simulink model "Q5"  (R2017b)
settings: Solver=VariableStepAuto  StartTime=0.0  StopTime=50  RelTol=1e-3
libraries: simulink x2
settings Model: Creator=HeMaTshop  LastModifiedBy=HeMaTshop

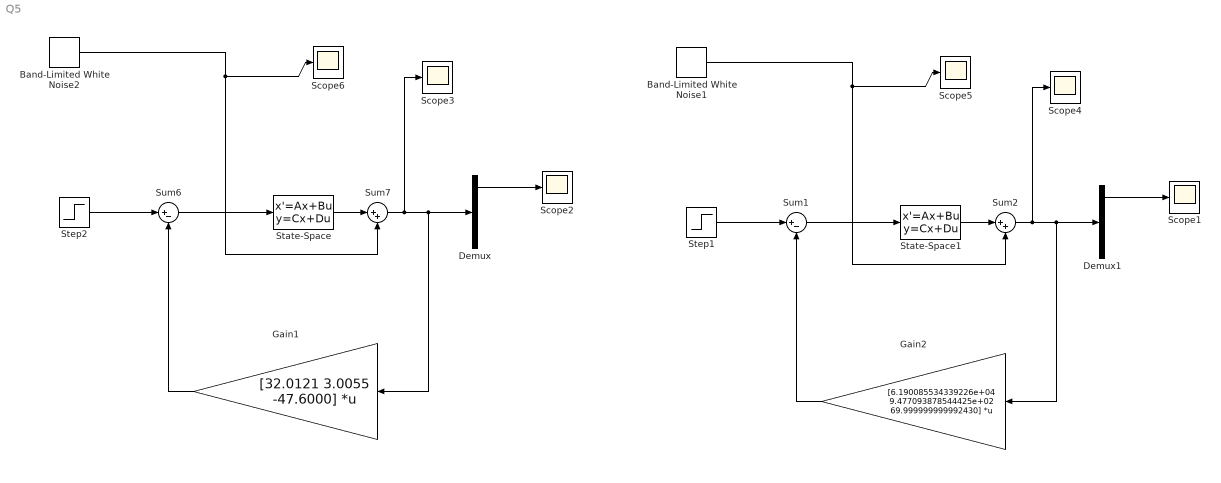
== system Q5 ==
  Band-Limited White Noise1 : simulink/Sources/Band-Limited White Noise  Cov=[0.001]  Ts=1  seed=[23341]
  Band-Limited White Noise2 : simulink/Sources/Band-Limited White Noise  Cov=[0.001]  Ts=1  seed=[23341]
  Demux : Demux  Outputs=3
  Demux1 : Demux  Outputs=3
  Gain1 : Gain  Gain="[32.0121    3.0055  -47.6000]"  Multiplication=Matrix(K*u)
  Gain2 : Gain  Gain="[6.190085534339226e+04    9.477093878544425e+02  69.999999999992430]"  Multiplication=Matrix(K*u)
  Scope{1..6} (6 alike) : Scope
  State-Space : StateSpace  A=[0 1 0;9.8/0.03 0 24.8656;0 0 -250]  B=[0;0;5]  C=eye(3)  D=[0;0;0]  InitialCondition=0
  State-Space1 : StateSpace  A=[0 1 0;9.8/0.03 0 24.8656;0 0 -250]  B=[0;0;5]  C=eye(3)  D=[0;0;0]  InitialCondition=0
  Step1 : Step  Time=0  SampleTime=0
  Step2 : Step  Time=0  SampleTime=0
  Sum1 : Sum  Inputs=|+-
  Sum2 : Sum  Inputs=|++
  Sum6 : Sum  Inputs=|+-
  Sum7 : Sum  Inputs=|++
  wires:
  Sum7/1 -> Scope3/1, Gain1/1, Demux/1
  Gain1/1 -> Sum6/2
  Demux/1 -> Scope2/1
  Step2/1 -> Sum6/1
  Band-Limited White Noise2/1 -> Scope6/1, Sum7/2
  State-Space/1 -> Sum7/1
  Sum6/1 -> State-Space/1
  State-Space1/1 -> Sum2/1
  Sum1/1 -> State-Space1/1
  Band-Limited White Noise1/1 -> Scope5/1, Sum2/2
  Sum2/1 -> Scope4/1, Gain2/1, Demux1/1
  Gain2/1 -> Sum1/2
  Demux1/1 -> Scope1/1
  Step1/1 -> Sum1/1
